simulink model "Airbag"  (R2023a)
settings: Solver=VariableStepAuto  StartTime=0.0  StopTime=10.0  RelTol=1e-3
settings Model: Creator=gurus  LastModifiedBy=gurus

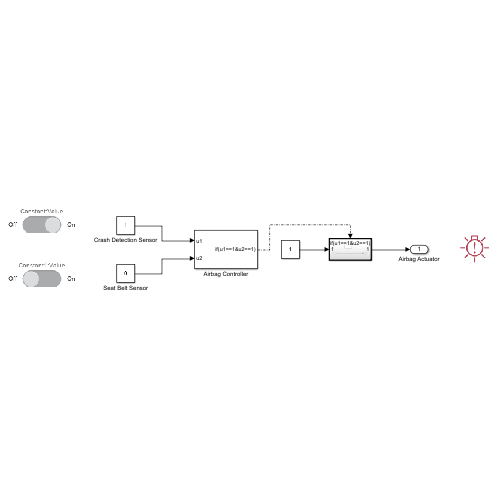
[thumbnail: Simulink's stored preview of the top-level diagram]
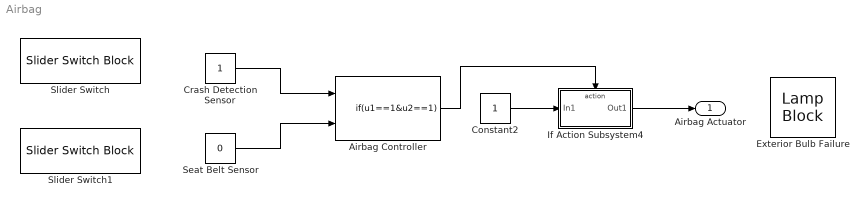
== system Airbag ==
  Airbag Controller : If  NumInputs=2  IfExpression=u1==1&u2==1  ShowElse=off
  Constant2 : Constant
  Crash Detection Sensor : Constant
  Exterior Bulb Failure : LampBlock  LabelPosition=Hide  Icon=ExteriorBulbFailure
  If Action Subsystem4 : Subsystem  TreatAsAtomicUnit=on
  Seat Belt Sensor : Constant  Value=0
  Slider Switch : SliderSwitchBlock
      settings: Values={{'Off', 'On'}, [0 1]}
  Slider Switch1 : SliderSwitchBlock
      settings: Values={{'Off', 'On'}, [0 1]}
  Airbag Actuator : Outport
  wires:
  Crash Detection Sensor/1 -> Airbag Controller/1
  Seat Belt Sensor/1 -> Airbag Controller/2
  Airbag Controller/1 -> If Action Subsystem4/Action
  Constant2/1 -> If Action Subsystem4/1(In1)
  If Action Subsystem4/1(Out1) -> Airbag Actuator/1

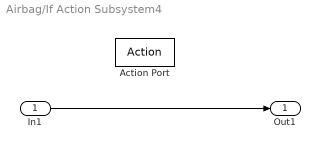
== system Airbag/If Action Subsystem4 ==
  In1 : Inport
  Action Port : ActionPort  ActionPortLabel=if(u1==1&u2==1)
  Out1 : Outport
  wires:
  In1/1 -> Out1/1
